simulink model "observer_test"  (R2021b)
settings: Solver=VariableStepAuto  StartTime=0.0  StopTime=5  RelTol=1e-3
model workspace (MAT data in the model file):
  a = 0
values from neighbouring files (symbols this model uses):
  P = [Dd ... (first row only)    [CASU2_2.m]    (also in chernovik.m = [B)
  Q = [G + Dd*K, zeros(3, 3);      L*C, G+Dd*K-L*C]    [CASU2_2.m]    (also in chernovik.m = [A + B*K, [0, 0, 0; 0, 0, 0; 0, 0, 0];      A + B*K + L*C, -)
  R = [1, 0, 0, 0, 0, 0 ... (first row only)    [CASU2_2.m]    (also in chernovik.m = [1, 0, 0, 1, 0, 0])
settings Model: Creator=s-dzu  LastModifiedBy=s-dzu

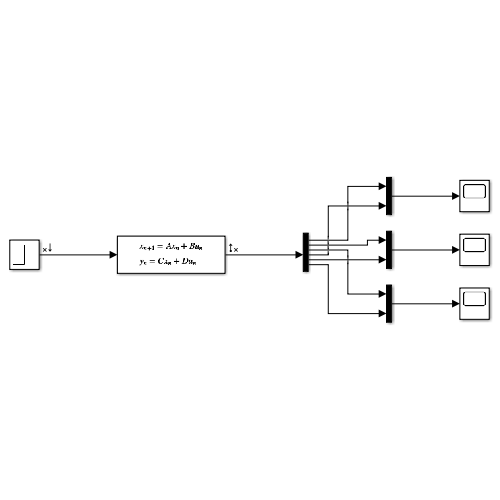
[thumbnail: Simulink's stored preview of the top-level diagram]
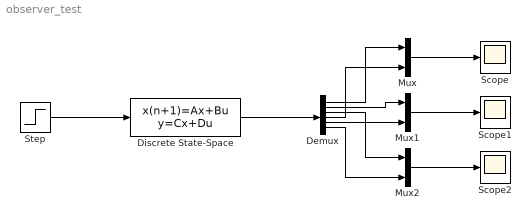
== system observer_test ==
  Demux : Demux  Outputs=6
  Discrete State-Space : DiscreteStateSpace  A=Q  B=P  C=R  D=[0;0;0;0;0;0]  InitialCondition=[1;1;1;2;2;2]  SampleTime=-1
  Mux : Mux  Inputs=2
  Mux1 : Mux  Inputs=2
  Mux2 : Mux  Inputs=2
  Scope : Scope
  Scope1 : Scope
  Scope2 : Scope
  Step : Step  SampleTime=0
  wires:
  Discrete State-Space/1 -> Demux/1
  Step/1 -> Discrete State-Space/1
  Mux/1 -> Scope/1
  Mux1/1 -> Scope1/1
  Mux2/1 -> Scope2/1
  Demux/1 -> Mux/1
  Demux/3 -> Mux2/1
  Demux/2 -> Mux1/1
  Demux/4 -> Mux/2
  Demux/6 -> Mux2/2
  Demux/5 -> Mux1/2
